simulink model "Quadrotor_14_step4_disc_section1_done"  (Simulink 7.6)
settings: Solver=ode45  StartTime=0.0  StopTime=800  RelTol=1e-3
undefined symbols (not defined in the file): STARMAC, uav_utilities
libraries: simulink x25, aero_sim_lib x8
(part 2 of 2)

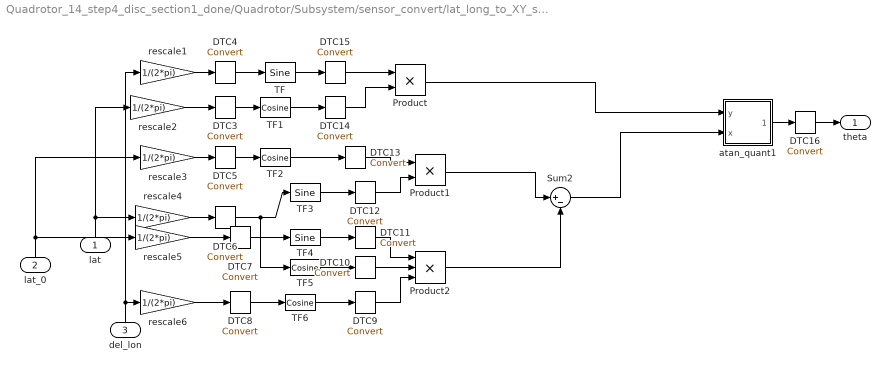
== system Quadrotor_14_step4_disc_section1_done/Quadrotor/Subsystem/sensor_convert/lat_long_to_XY_subsys/angle ==
  lat : Inport
  lat_0 : Inport  Port=2
  del_lon : Inport  Port=3
  DTC{3..16} (14 alike) : DataTypeConversion
  Product : Product  OutDataTypeStr=fixdt(1,128,58)  RndMeth=Zero
  Product1 : Product  OutDataTypeStr=fixdt(1,128,58)  RndMeth=Zero
  Product2 : Product  Inputs=3  OutDataTypeStr=fixdt(1,128,58)  RndMeth=Zero
  Sum2 : Sum  Inputs=|+-
  TF : simulink/Lookup Tables/Sine  SystemSampleTime=-1  Formula=sin(2*pi*u)  NumDataPoints=(2^7)+1  OutputWordLength=32
  TF{1..2,5..6} (4 alike) : simulink/Lookup Tables/Cosine  SystemSampleTime=-1  Formula=cos(2*pi*u)  NumDataPoints=(2^7)+1  OutputWordLength=32
  TF3 : simulink/Lookup Tables/Sine  SystemSampleTime=-1  Formula=sin(2*pi*u)  NumDataPoints=(2^7)+1  OutputWordLength=32
  TF4 : simulink/Lookup Tables/Sine  SystemSampleTime=-1  Formula=sin(2*pi*u)  NumDataPoints=(2^7)+1  OutputWordLength=32
  atan_quant1 : Subsystem
  rescale{1..6} (6 alike) : Gain  Gain=1/(2*pi)
  theta : Outport
  wires:
  TF/1 -> DTC15/1
  TF1/1 -> DTC14/1
  Product1/1 -> Sum2/1
  Product2/1 -> Sum2/2
  TF2/1 -> DTC13/1
  TF3/1 -> DTC12/1
  TF4/1 -> DTC11/1
  TF5/1 -> DTC10/1
  TF6/1 -> DTC9/1
  Product/1 -> atan_quant1/1(y)
  lat/1 -> rescale2/1, rescale4/1
  lat_0/1 -> rescale3/1, rescale5/1
  del_lon/1 -> rescale1/1, rescale6/1
  atan_quant1/1(atan2) -> DTC16/1
  rescale1/1 -> DTC4/1
  DTC4/1 -> TF/1
  rescale2/1 -> DTC3/1
  DTC3/1 -> TF1/1
  rescale3/1 -> DTC5/1
  DTC5/1 -> TF2/1
  rescale4/1 -> DTC6/1
  rescale5/1 -> DTC7/1
  DTC7/1 -> TF4/1
  DTC6/1 -> TF5/1, TF3/1
  rescale6/1 -> DTC8/1
  DTC8/1 -> TF6/1
  DTC9/1 -> Product2/3
  DTC10/1 -> Product2/2
  DTC11/1 -> Product2/1
  DTC12/1 -> Product1/2
  DTC13/1 -> Product1/1
  DTC14/1 -> Product/2
  DTC15/1 -> Product/1
  Sum2/1 -> atan_quant1/2(x)
  DTC16/1 -> theta/1

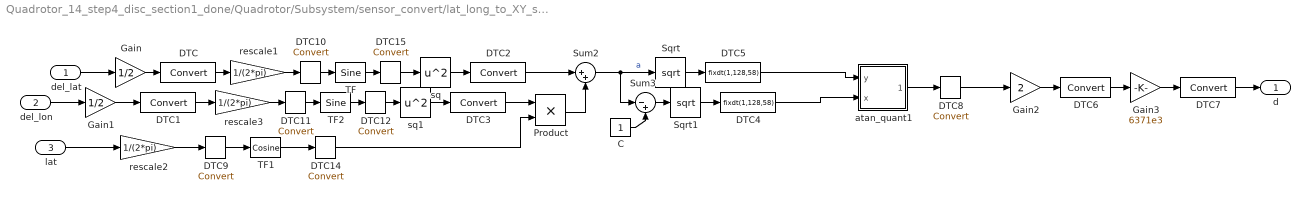
== system Quadrotor_14_step4_disc_section1_done/Quadrotor/Subsystem/sensor_convert/lat_long_to_XY_subsys/dist ==
  del_lat : Inport
  del_lon : Inport  Port=2
  lat : Inport  Port=3
  C : Constant
  DTC{,1..3,6..12,14..15} (13 alike) : DataTypeConversion
  DTC4 : DataTypeConversion  OutDataTypeStr=fixdt(1,128,58)  LockScale=on
  DTC5 : DataTypeConversion  OutDataTypeStr=fixdt(1,128,58)  LockScale=on
  Gain : Gain  Gain=1/2
  Gain1 : Gain  Gain=1/2
  Gain2 : Gain  Gain=2
  Gain3 : Gain  Gain=6371e3
  Product : Product  RndMeth=Zero
  Sqrt : Sqrt  SaturateOnIntegerOverflow=on
  Sqrt1 : Sqrt  SaturateOnIntegerOverflow=on
  Sum2 : Sum  Inputs=|++
  Sum3 : Sum  Inputs=|-+
  TF : simulink/Lookup Tables/Sine  SystemSampleTime=-1  Formula=sin(2*pi*u)  NumDataPoints=(2^7)+1  OutputWordLength=32
  TF1 : simulink/Lookup Tables/Cosine  SystemSampleTime=-1  Formula=cos(2*pi*u)  NumDataPoints=(2^7)+1  OutputWordLength=32
  TF2 : simulink/Lookup Tables/Sine  SystemSampleTime=-1  Formula=sin(2*pi*u)  NumDataPoints=(2^7)+1  OutputWordLength=32
  atan_quant1 : Subsystem
  rescale1 : Gain  Gain=1/(2*pi)
  rescale2 : Gain  Gain=1/(2*pi)
  rescale3 : Gain  Gain=1/(2*pi)
  sq : Math  Operator=square  SaturateOnIntegerOverflow=on
  sq1 : Math  Operator=square  SaturateOnIntegerOverflow=on
  d : Outport
  wires:
  Gain/1 -> DTC/1
  Gain1/1 -> DTC1/1
  sq/1 -> DTC2/1
  sq1/1 -> DTC3/1
  Sum2/1 -> Sum3/1, Sqrt/1  "a"
  C/1 -> Sum3/2
  Sum3/1 -> Sqrt1/1
  Sqrt/1 -> DTC5/1
  Sqrt1/1 -> DTC4/1
  atan_quant1/1(atan2) -> DTC8/1
  Gain2/1 -> DTC6/1
  del_lat/1 -> Gain/1
  Gain3/1 -> DTC7/1
  del_lon/1 -> Gain1/1
  DTC2/1 -> Sum2/1
  DTC6/1 -> Gain3/1
  DTC7/1 -> d/1
  TF/1 -> DTC15/1
  TF1/1 -> DTC14/1
  rescale1/1 -> DTC10/1
  DTC10/1 -> TF/1
  rescale2/1 -> DTC9/1
  DTC9/1 -> TF1/1
  DTC/1 -> rescale1/1
  DTC15/1 -> sq/1
  TF2/1 -> DTC12/1
  rescale3/1 -> DTC11/1
  DTC11/1 -> TF2/1
  DTC1/1 -> rescale3/1
  DTC12/1 -> sq1/1
  lat/1 -> rescale2/1
  DTC14/1 -> Product/2
  DTC3/1 -> Product/1
  Product/1 -> Sum2/2
  DTC5/1 -> atan_quant1/1(y)
  DTC4/1 -> atan_quant1/2(x)
  DTC8/1 -> Gain2/1

== system Quadrotor_14_step4_disc_section1_done/Quadrotor/Subsystem/sensor_convert/lat_long_to_XY_subsys/lat_lon_0 ==
  lat : Inport
  lon : Inport  Port=2
  Constant : Constant
  Demux : Demux  Outputs=2
  Mux : Mux  Inputs=2
  Mux1 : Mux  Inputs=2
  Switch : Switch  Criteria=u2 ~= 0
  indicator : UnitDelay  SampleTime=-1
  lat_0_d : UnitDelay  SampleTime=-1
  lon_0_d : UnitDelay  SampleTime=-1
  lat_0 : Outport
  lon_0 : Outport  Port=2
  wires:
  Constant/1 -> indicator/1
  indicator/1 -> Switch/2
  Mux/1 -> Switch/3
  lat_0_d/1 -> Mux1/1
  lon_0_d/1 -> Mux1/2
  Mux1/1 -> Switch/1
  Switch/1 -> Demux/1
  Demux/1 -> lat_0_d/1, lat_0/1
  Demux/2 -> lon_0_d/1, lon_0/1
  lat/1 -> Mux/1
  lon/1 -> Mux/2

== system Quadrotor_14_step4_disc_section1_done/Quadrotor/plant_dynamics/starmac_blade_flapping_effects/starmac_body_moments/CrossProduct(AXB) ==
  A : Inport
  B : Inport  Port=2
  Fcn : Fcn  Expr=u[2]*u[6]-u[3]*u[5]
  Fcn1 : Fcn  Expr=u[3]*u[4]-u[1]*u[6]
  Fcn2 : Fcn  Expr=u[1]*u[5]-u[2]*u[4]
  Mux : Mux  Inputs=2
  Mux1 : Mux  Inputs=3
  Out : Outport
  wires:
  Mux1/1 -> Out/1
  Fcn2/1 -> Mux1/3
  Fcn1/1 -> Mux1/2
  Fcn/1 -> Mux1/1
  Mux/1 -> Fcn2/1, Fcn1/1, Fcn/1
  B/1 -> Mux/2
  A/1 -> Mux/1

== system Quadrotor_14_step4_disc_section1_done/Quadrotor/plant_dynamics/starmac_blade_flapping_effects/starmac_body_moments/CrossProduct(AXB)1 ==
  A : Inport
  B : Inport  Port=2
  Fcn : Fcn  Expr=u[2]*u[6]-u[3]*u[5]
  Fcn1 : Fcn  Expr=u[3]*u[4]-u[1]*u[6]
  Fcn2 : Fcn  Expr=u[1]*u[5]-u[2]*u[4]
  Mux : Mux  Inputs=2
  Mux1 : Mux  Inputs=3
  Out : Outport
  wires:
  A/1 -> Mux/1
  B/1 -> Mux/2
  Mux/1 -> Fcn/1, Fcn1/1, Fcn2/1
  Fcn/1 -> Mux1/1
  Fcn1/1 -> Mux1/2
  Fcn2/1 -> Mux1/3
  Mux1/1 -> Out/1

== system Quadrotor_14_step4_disc_section1_done/Quadrotor/plant_dynamics/starmac_blade_flapping_effects/starmac_body_moments/CrossProduct(AXB)2 ==
  A : Inport
  B : Inport  Port=2
  Fcn : Fcn  Expr=u[2]*u[6]-u[3]*u[5]
  Fcn1 : Fcn  Expr=u[3]*u[4]-u[1]*u[6]
  Fcn2 : Fcn  Expr=u[1]*u[5]-u[2]*u[4]
  Mux : Mux  Inputs=2
  Mux1 : Mux  Inputs=3
  Out : Outport
  wires:
  Mux1/1 -> Out/1
  Fcn2/1 -> Mux1/3
  Fcn1/1 -> Mux1/2
  Fcn/1 -> Mux1/1
  Mux/1 -> Fcn2/1, Fcn1/1, Fcn/1
  B/1 -> Mux/2
  A/1 -> Mux/1

== system Quadrotor_14_step4_disc_section1_done/Quadrotor/plant_dynamics/starmac_blade_flapping_effects/starmac_body_moments/CrossProduct(AXB)3 ==
  A : Inport
  B : Inport  Port=2
  Fcn : Fcn  Expr=u[2]*u[6]-u[3]*u[5]
  Fcn1 : Fcn  Expr=u[3]*u[4]-u[1]*u[6]
  Fcn2 : Fcn  Expr=u[1]*u[5]-u[2]*u[4]
  Mux : Mux  Inputs=2
  Mux1 : Mux  Inputs=3
  Out : Outport
  wires:
  A/1 -> Mux/1
  B/1 -> Mux/2
  Mux/1 -> Fcn/1, Fcn1/1, Fcn2/1
  Fcn/1 -> Mux1/1
  Fcn1/1 -> Mux1/2
  Fcn2/1 -> Mux1/3
  Mux1/1 -> Out/1

== system Quadrotor_14_step4_disc_section1_done/Quadrotor/plant_dynamics/starmac_blade_flapping_effects/starmac_body_moments/Motor Thrust to Torques ==
  Thrusts : Inport
  Demux : Demux
  Gain1 : Gain  Gain=K_torque
  torque 1 : Outport
  torque 2 : Outport  Port=2
  torque 3 : Outport  Port=3
  torque 4 : Outport  Port=4
  wires:
  Demux/4 -> torque 4/1
  Demux/3 -> torque 3/1
  Demux/2 -> torque 2/1
  Demux/1 -> torque 1/1
  Gain1/1 -> Demux/1
  Thrusts/1 -> Gain1/1

== system Quadrotor_14_step4_disc_section1_done/Quadrotor/Subsystem/Outer_Loop/body_to_inertial/inertial_vel_and pos_est/DT_integrator ==
  Ab : Inport
  DTC : DataTypeConversion
  Sum : Sum  Inputs=++|
  Sum1 : Sum  Inputs=|++
  negate : Gain  Gain=.5*Ts
  u_delay : UnitDelay  SampleTime=-1
  u_delay1 : UnitDelay  SampleTime=-1
  Vb : Outport
  wires:
  Ab/1 -> u_delay/1, Sum/2
  u_delay/1 -> Sum/1
  Sum/1 -> negate/1
  negate/1 -> DTC/1
  Sum1/1 -> u_delay1/1, Vb/1
  u_delay1/1 -> Sum1/2
  DTC/1 -> Sum1/1

== system Quadrotor_14_step4_disc_section1_done/Quadrotor/Subsystem/Outer_Loop/body_to_inertial/inertial_vel_and pos_est/DT_integrator1 ==
  Vb : Inport
  DTC : DataTypeConversion
  Sum : Sum  Inputs=++|
  Sum1 : Sum  Inputs=|++
  negate : Gain  Gain=.5*Ts
  u_delay : UnitDelay  SampleTime=-1
  u_delay1 : UnitDelay  SampleTime=-1
  Xb : Outport  PortDimensions=[3]
  wires:
  u_delay1/1 -> Sum1/2
  Sum1/1 -> Xb/1, u_delay1/1
  negate/1 -> DTC/1
  Sum/1 -> negate/1
  u_delay/1 -> Sum/1
  Vb/1 -> Sum/2, u_delay/1
  DTC/1 -> Sum1/1

== system Quadrotor_14_step4_disc_section1_done/Quadrotor/Subsystem/sensor_convert/lat_long_to_XY_subsys/angle/atan_quant1 ==
  y : Inport
  x : Inport  Port=2
  Compare To Zero : simulink/Logic and Bit Operations/Compare To Zero  SystemSampleTime=-1  relop=<  LogicOutDataTypeMode=uint8
  Compare To Zero1 : simulink/Logic and Bit Operations/Compare To Zero  SystemSampleTime=-1  relop=<  LogicOutDataTypeMode=uint8
  Constant : Constant  Value=pi  OutDataTypeStr=Inherit: Inherit via back propagation
  Data Type Conversion : DataTypeConversion  OutDataTypeStr=fixdt(1,32,26)  SaturateOnIntegerOverflow=on
  Data Type Conversion1 : DataTypeConversion  OutDataTypeStr=fixdt(1,32,29)
  Divide : Product  Inputs=*/  SaturateOnIntegerOverflow=on  OutDataTypeStr=Inherit: Same as first input
  Sum : Sum  Inputs=-+|  OutDataTypeStr=Inherit: Inherit via back propagation
  Sum1 : Sum  Inputs=++|  OutDataTypeStr=Inherit: Inherit via back propagation
  Switch1 : Switch  Criteria=u2 ~= 0  OutDataTypeStr=Inherit: Inherit via back propagation
  Switch3 : Switch  Criteria=u2 ~= 0  OutDataTypeStr=Inherit: Inherit via back propagation
  TF1 : Lookup  InputValues=fi([-10:.8:10], 1, 32, 26)  Table=fi([ -pi/2 atan([-(10-.8):.8:(10-.8)]) pi/2 ], 1, 32, 29)  LookUpMeth=Interpolation-Use End Values  OutDataTypeStr=fixdt(1,32,29)
  atan2 : Outport
  wires:
  y/1 -> Divide/1, Compare To Zero/1
  x/1 -> Divide/2, Compare To Zero1/1
  Divide/1 -> Data Type Conversion/1
  Switch3/1 -> Switch1/1
  TF1/1 -> Data Type Conversion1/1
  Constant/1 -> Sum1/1, Sum/1
  Sum/1 -> Switch3/1
  Sum1/1 -> Switch3/3
  Compare To Zero/1 -> Switch3/2
  Compare To Zero1/1 -> Switch1/2
  Data Type Conversion/1 -> TF1/1
  Data Type Conversion1/1 -> Sum/2, Sum1/2, Switch1/3
  Switch1/1 -> atan2/1

== system Quadrotor_14_step4_disc_section1_done/Quadrotor/Subsystem/sensor_convert/lat_long_to_XY_subsys/dist/atan_quant1 ==
  y : Inport
  x : Inport  Port=2
  Compare To Zero : simulink/Logic and Bit Operations/Compare To Zero  SystemSampleTime=-1  relop=<  LogicOutDataTypeMode=uint8
  Compare To Zero1 : simulink/Logic and Bit Operations/Compare To Zero  SystemSampleTime=-1  relop=<  LogicOutDataTypeMode=uint8
  Constant : Constant  Value=pi  OutDataTypeStr=Inherit: Inherit via back propagation
  Data Type Conversion : DataTypeConversion  OutDataTypeStr=fixdt(1,32,26)  SaturateOnIntegerOverflow=on
  Data Type Conversion1 : DataTypeConversion  OutDataTypeStr=fixdt(1,32,29)
  Divide : Product  Inputs=*/  SaturateOnIntegerOverflow=on  OutDataTypeStr=Inherit: Same as first input
  Sum : Sum  Inputs=-+|  OutDataTypeStr=Inherit: Inherit via back propagation
  Sum1 : Sum  Inputs=++|  OutDataTypeStr=Inherit: Inherit via back propagation
  Switch1 : Switch  Criteria=u2 ~= 0  OutDataTypeStr=Inherit: Inherit via back propagation
  Switch3 : Switch  Criteria=u2 ~= 0  OutDataTypeStr=Inherit: Inherit via back propagation
  TF1 : Lookup  InputValues=fi([-10:.8:10], 1, 32, 26)  Table=fi([ -pi/2 atan([-(10-.8):.8:(10-.8)]) pi/2 ], 1, 32, 29)  LookUpMeth=Interpolation-Use End Values  OutDataTypeStr=fixdt(1,32,29)
  atan2 : Outport
  wires:
  y/1 -> Divide/1, Compare To Zero/1
  x/1 -> Divide/2, Compare To Zero1/1
  Divide/1 -> Data Type Conversion/1
  Switch3/1 -> Switch1/1
  TF1/1 -> Data Type Conversion1/1
  Constant/1 -> Sum1/1, Sum/1
  Sum/1 -> Switch3/1
  Sum1/1 -> Switch3/3
  Compare To Zero/1 -> Switch3/2
  Compare To Zero1/1 -> Switch1/2
  Data Type Conversion/1 -> TF1/1
  Data Type Conversion1/1 -> Sum/2, Sum1/2, Switch1/3
  Switch1/1 -> atan2/1

== matlab function Quadrotor/GPS/XY-to-lat_long/XY-to-lat_long ==
  data: XY input double size=[2]; lat output double; lon output double; lat_0 parameter double; lon_0 parameter double
function [lat,lon] = fcn(XY, lat_0, lon_0)
%Convert inertial X position and Inertial Y position to latitude and
%longitude
    R = 6371e3;          %Earth's Radius meters
    X = XY(1);           %Inertial X position meters
    Y = XY(2);           %Inertial Y position meters
    lat_0 = lat_0*pi/180;
    lon_0 = lon_0*pi/180;
    theta = atan2(Y,X);  %Radians
    d = sqrt(X^2 + Y^2); %Distance from start point (lat_0, lon_0)
    alpha = d/R;
    lat = lat_0 + alpha*cos(theta);
    if abs(theta) == pi/2
        q = cos(lat_0);
    else
        tmp = log(tan((lat/2) + (pi/4))/tan((lat_0/2) + (pi/4)));
        q = alpha*cos(theta)/tmp;
    end
    del_lon = alpha*sin(theta)/q;
    lon = mod((lon_0 + del_lon + pi),2*pi)-pi;
    lat = (180/pi)*lat; %degrees
    lon = (180/pi)*lon; %degrees
    lat = 1e7*lat; %1e-7 degrees
    lon = 1e7*lon; %1e-7 degrees
